simulink library "xpclib"  (Simulink 6.0)
settings: Solver=ode45  SolverMode=SingleTasking  StartTime=0.0  StopTime=10.0  RelTol=1e-3
values from neighbouring files (symbols this model uses):
  base = get_param( gcb, 'base' )    [maddiamondmm.m]    (also in maddiamondmm32.m; maddiamondmm32frame.m; maddsmm16at.m; malaim16.m = hex2dec(baseaddress(3:end)))
  data = ''    [mbwaudpmc.m]
  irq = params{3}    [mbaseserialmask.m]
  port = [0,1]    [canfifofilterutil.m]    (also in mbaseserialmask.m = str2num(get_param( gcb, 'port' )))
undefined symbols (not defined in the file or in its folder): CIO, devid, DIO24, genixlib, get, handlers, mbaseserialmask, mbwaudpmc, mdacbpcidas, mdiamondemeraldmask, mgenix, mmodemcontrol, mquamask, mrs232, msc150checks, mtargetboxleds, mtargetboxwatchdog, mxpccan, PCI, sizeof, vendid
libraries: xpclib x384, simulink x6
(part 5 of 7)

== system xpclib/RS232/Quatech/QSC-200/300 ==
  Modem Control : S-Function  InitFcn=mmodemcontrol(3)  FunctionName=modemcontrolqua  Parameters=slot, port, boardtype, rts, dtr, count  mask(QSC-200/300 Modem Control){port=1, rts=on, dtr=on, slot=-1}
      mask prompts: slot "PCI slot: (-1 for autosearch)"
      mask help:
      | QSC-200/300
      | Quatech
      | Modem Control
      mask init:
      | count = 0;
      | boardtype = 3;
      | [maskdisplay, count] = mmodemcontrol( 2, rts, dtr, boardtype, 0, 0 );
      | set_param( gcb, 'MaskDisplay', maskdisplay );
      mask Help: helpview(fullfile(docroot, 'mapfiles', 'xpc.map'), 'Quatech_MODEM_Control')
      mask StyleString: popup(1|2|3|4),checkbox,checkbox,edit
      mask Display: disp('QSC-200/300\nQuatech\nModem Control');port_label('input',1,'RTS');port_label('input',2,'DTR');
  Modem Status : S-Function  FunctionName=modemstatusqua  Parameters=slot, port, boardtype, cts, dsr, ring, dcd, count, sampletime  mask(Modem Status){port=1, cts=on, dsr=on, ring=on, dcd=on, sampletime=-1, slot=-1}
      mask prompts: ring "RI:"; slot "PCI slot: (-1 for autosearch)"
      mask help:
      | QSC-200/300
      | Quatech
      | Modem Status
      mask init:
      | count = 0;
      | boardtype = 3;
      | [maskdisplay, count] = mmodemstatus( 2, cts, dsr, ring, dcd, boardtype );
      | set_param( gcb, 'MaskDisplay', maskdisplay );
      mask Help: helpview(fullfile(docroot, 'mapfiles', 'xpc.map'), 'Quatech_MODEM_Status')
      mask StyleString: popup(1|2|3|4),checkbox,checkbox,checkbox,checkbox,edit,edit
      mask Display: disp('QSC-200/300\nQuatech\nModem Status');port_label('output',1,'CTS');port_label('output',2,'DSR');port_label('output',3,'RI');port_label('output',4,'DCD');
  QSC-200/300 Internal  blocks1 : Subsystem  PropExecContextAcrossSSBoundary=on
  "QSC-200/300 " : Subsystem  InitFcn=mquamask(3)  TreatAsAtomicUnit=on  PropExecContextAcrossSSBoundary=on  mask(RS422/485 Send Receive){group=Board Setup, port=1, irqnum=7, slot=-1, baud1=115200, parity1=None, ndata1=8, nstop1=1, fifomode1=64 deep, rlevel1=half full, onxmt1=None, xmtfifosize1=1024, xmtdatatype1=8 bit uint null terminated, rcvfifosize1=1024, rcvmaxread1=1024, rcvminread1=1, rcvusedelim1=on, rcvdelim1=13, rcvdatatype1=count+16 bit uint, rcvsampletime1=-1, baud2=115200, parity2=None, ndata2=8, nstop2=1, fifomode2=64 deep, rlevel2=half full, onxmt2=None, xmtfifosize2=1024, xmtdatatype2=8 bit uint null terminated, rcvfifosize2=1024, rcvmaxread2=1024, rcvminread2=1, rcvusedelim2=on, rcvdelim2=13, rcvdatatype2=count+16 bit uint, rcvsampletime2=-1, baud3=115200, parity3=None, ndata3=8, nstop3=1, fifomode3=64 deep, rlevel3=half full, onxmt3=None, xmtfifosize3=1024, xmtdatatype3=8 bit uint null terminated, rcvfifosize3=1024, rcvmaxread3=1024, rcvminread3=1, rcvusedelim3=on, rcvdelim3=13, rcvdatatype3=count+16 bit uint, rcvsampletime3=-1, buad4=115200, parity4=None, ndata4=8, nstop4=1, fifomode4=64 deep, rlevel4=half full, onxmt4=None, xmtfifosize4=1024, xmtdatatype4=8 bit uint null terminated, rcvfifosize4=1024, rcvmaxread4=1024, rcvminread4=1, rcvusedelim4=on, rcvdelim4=13, rcvdatatype4=count+16 bit uint, rcvsampletime4=-1}
      mask prompts: group "Parameter group:"; port "Port to modify:"; irqnum "IRQ number:"; baud1 "Baud rate:"; parity1 "Parity:"; ndata1 "Data bits:"; nstop1 "Stop bits:"; fifomode1 "Hardware fifo size:"; rlevel1 "Receive fifo interrupt level:"; onxmt1 "Assert on transmit:"; xmtfifosize1 "Transmit software fifo size:"; xmtdatatype1 "Transmit fifo data type:"; rcvfifosize1 "Receive software fifo size:"; rcvmaxread1 "Receive maximum read:"; rcvminread1 "Receive minimum read:"; rcvusedelim1 "Read to delimiter:"; rcvdelim1 "Delimiter:"; rcvdatatype1 "Receive data type:"; rcvsampletime1 "Receive SampleTime:"; baud2 "Baud rate:"; parity2 "Parity:"; ndata2 "Data bits:"; nstop2 "Stop bits:"; fifomode2 "Hardware fifo size:"; rlevel2 "Receive fifo interrupt level:"; onxmt2 "Assert on transmit:"; xmtfifosize2 "Transmit software fifo size:"; xmtdatatype2 "Transmit fifo data type:"; rcvfifosize2 "Receive software fifo size:"; rcvmaxread2 "Receive maximum read:"; rcvminread2 "Receive minimum read:"; rcvusedelim2 "Read to delimiter:"; rcvdelim2 "Delimiter:"; rcvdatatype2 "Receive data type:"; rcvsampletime2 "Receive SampleTime:"; baud3 "Baud rate:"; parity3 "Parity:"; ndata3 "Data bits:"; nstop3 "Stop bits:"; fifomode3 "Hardware fifo size:"; rlevel3 "Receive fifo interrupt level:"; onxmt3 "Assert on transmit:"; xmtfifosize3 "Transmit software fifo size:"; xmtdatatype3 "Transmit fifo data type:"; rcvfifosize3 "Receive software fifo size:"; rcvmaxread3 "Receive maximum read:"; rcvminread3 "Receive minimum read:"; rcvusedelim3 "Read to delimiter:"; rcvdelim3 "Delimiter:"; rcvdatatype3 "Receive data type:"; rcvsampletime3 "Receive SampleTime:"; buad4 "Baud rate:"; parity4 "Parity:"; ndata4 "Data bits:"; nstop4 "Stop bits:"; fifomode4 "Hardware fifo size:"; rlevel4 "Receive fifo interrupt level:"; onxmt4 "Assert on transmit:"; xmtfifosize4 "Transmit software fifo size:"; xmtdatatype4 "Transmit fifo data type:"; rcvfifosize4 "Receive software fifo size:"; rcvmaxread4 "Receive maximum read:"; rcvminread4 "Receive minimum read:"; rcvusedelim4 "Read to delimiter:"; rcvdelim4 "Delimiter:"; rcvdatatype4 "Receive data type:"; rcvsampletime4 "Receive SampleTime:"
      mask help:
      | QSC-200/300
      | Quatech
      | RS422/485 Send Receive Subsystem
      mask init:
      | brdslot = slot;
      | mqua2mask( 1, 4 );
      mask Help: helpview(fullfile(docroot, 'mapfiles', 'xpc.map'), 'Quatech_Subsystem')
      mask StyleString: popup(Board Setup|Basic Setup|Transmit Setup|Receive Setup),popup(1|2|3|4),edit,edit,popup(921600|460800|230400|115200|57600|38400|19200|9600|4800|2400|1200|600|300|110),popup(None|Even|Odd|Mark|Space),popup(5|6|7|8),popup(1|2),popup(64 deep|16 deep|1 deep),popup(1|quarter full|half full|almost full),popup(None|RTS|DTR),edit,popup(count+32 bit int|count+32 bit uint|count+16 bit int|count+16 bit uint|8 bit int null terminated|8 bit uint null terminated),edit,edit,edit,checkbox,edit,popup(count+32 bit int|count+32 bit uint|count+16 bit int|count+16 bit uint|8 bit int null terminated|8 bit uint null terminated),edit,popup(921600|460800|230400|115200|57600|38400|19200|9600|4800|2400|1200|600|300|110),popup(None|Even|Odd|Mark|Space),popup(5|6|7|8),popup(1|2),popup(64 deep|16 deep|1 deep),popup(1|quarter full|half full|almost full),popup(None|RTS|DTR),edit,popup(count+32 bit int|count+32 bit uint|count+16 bit int|count+16 bit uint|8 bit int null terminated|8 bit uint null terminated),edit,edit,edit,checkbox,edit,popup(count+32 bit int|count+32 bit uint|count+16 bit int|count+16 bit uint|8 bit int null terminated|8 bit uint null terminated),edit,popup(921600|460800|230400|115200|57600|38400|19200|9600|4800|2400|1200|600|300|110),popup(None|Even|Odd|Mark|Space),popup(5|6|7|8),popup(1|2),popup(64 deep|16 deep|1 deep),popup(1|quarter full|half full|almost full),popup(None|RTS|DTR),edit,popup(count+32 bit int|count+32 bit uint|count+16 bit int|count+16 bit uint|8 bit int null terminated|8 bit uint null terminated),edit,edit,edit,checkbox,edit,popup(count+32 bit int|count+32 bit uint|count+16 bit int|count+16 bit uint|8 bit int null terminated|8 bit uint null terminated),edit,popup(921600|460800|230400|115200|57600|38400|19200|9600|4800|2400|1200|600|300|110),popup(None|Even|Odd|Mark|Space),popup(5|6|7|8),popup(1|2),popup(64 deep|16 deep|1 deep),popup(1|quarter full|half full|almost full),popup(None|RTS|DTR),edit,popup(count+32 bit int|count+32 bit uint|count+16 bit int|count+16 bit uint|8 bit int null terminated|8 bit uint null terminated),edit,edit,edit,checkbox,edit,popup(count+32 bit int|count+32 bit uint|count+16 bit int|count+16 bit uint|8 bit int null terminated|8 bit uint null terminated),edit
      mask CallbackString:
      | mquamask( 2, 4 );
      | |mquamask( 2, 4 );||||||||||||||||||||||||||||||||||||||||||||||||||||||||||||||||||
      mask Display:
      | disp('QSC-200/300\n\nRS422/485\n\nSend Receive');
      | port_label( 'input', 1, 'XMT1' );
      | port_label( 'input', 2, 'XMT2' );
      | port_label( 'input', 3, 'XMT3' );
      | port_label( 'input', 4, 'XMT4' );
      | port_label( 'output', 1, 'RCV1' );
      | port_label( 'output', 2, 'RCV2' );
      | port_label( 'output', 3, 'RCV3' );
      | port_label( 'output', 4, 'RCV4' );

== system xpclib/RS232/Synchronous Mode/Send & Receive  ==
  In1 : Inport  LatchInput=off
  S-Function : S-Function  FunctionName=rs232_sendrec  Parameters=port,formatsend,formatrec,numb,ts
  Out1 : Outport
  wires:
  In1/1 -> S-Function/1
  S-Function/1 -> Out1/1

== system xpclib/CAN/Softing/CAN-AC2-104 SJA 1000/FIFO Mode ==
  "FIFO Read " : S-Function  FunctionName=canac2pcireceivef  Parameters=board, depth, status, sampletime  mask(canac2104readfifo){board=1, depth=1, status=off, sampletime=0.001}
      mask prompts: depth "FIFO read depth:"; status "Show status output port"; sampletime "Sample time:"
      mask help:
      | Softing
      | CAN-AC2-104
      | with SJA1000
      mask Help: helpview(fullfile(docroot, 'mapfiles', 'xpc.map'), 'Softing_CAN-AC2-104-SJA-1000_FIFO-Read')
      mask StyleString: popup(1|2|3),edit,checkbox,edit
      mask Display: disp(['CAN-AC2-104 B',num2str(board),'\nFIFO mode\nRead'])
  "FIFO Read Filter " : xpclib/CAN/Softing/CAN-AC2-PCI SJA 1000/FIFO Mode/FIFO Read Filter   portin=Any  direction=Exclude  ident=[]  identsel=Exclude
  "FIFO Read RCV Level " : S-Function  FunctionName=canac2readrcvfifolevel  Parameters=board, sampletime  mask(canac2readrcvfifolevel){board=1, sampletime=0.001}
      mask prompts: sampletime "Sample time:"
      mask help:
      | Softing
      | CAN-AC2-104
      | with SJA1000
      mask Help: helpview(fullfile(docroot, 'mapfiles', 'xpc.map'), 'Softing_CAN-AC2-104-SJA-1000_FIFO-Read-RCV-Level')
      mask StyleString: popup(1|2|3),edit
      mask Display: disp(['CAN-AC2-104 B',num2str(board),'\nFIFO mode\nRCV FIFO level'])
  "FIFO Read XMT Level " : S-Function  FunctionName=canac2readxmtfifolevel  Parameters=board, sampletime  mask(canac2readxmtfifolevel){board=1, sampletime=0.001}
      mask prompts: sampletime "Sample time:"
      mask help:
      | Softing
      | CAN-AC2-104
      | with SJA1000
      mask Help: helpview(fullfile(docroot, 'mapfiles', 'xpc.map'), 'Softing_CAN-AC2-104-SJA-1000_FIFO-Read-XMT-Level')
      mask StyleString: popup(1|2|3),edit
      mask Display: disp(['CAN-AC2-104 B',num2str(board),'\nFIFO mode\nXMT FIFO level'])
  "FIFO Reset RCV " : S-Function  FunctionName=canac2resetrcvfifo  Parameters=board, sampletime  mask(canac2resetrcvfifo){board=1, sampletime=0.001}
      mask prompts: sampletime "Sample time:"
      mask help:
      | Softing
      | CAN-AC2-104
      | with SJA1000
      mask Help: helpview(fullfile(docroot, 'mapfiles', 'xpc.map'), 'Softing_CAN-AC2-104-SJA-1000_FIFO-Reset-RCV')
      mask StyleString: popup(1|2|3),edit
      mask Display: disp(['CAN-AC2-104 B',num2str(board),'\nFIFO mode\nReset RCV FIFO'])
  "FIFO Reset XMT " : S-Function  FunctionName=canac2resetxmtfifo  Parameters=board, sampletime  mask(canac2resetxmtfifo){board=1, sampletime=0.001}
      mask prompts: sampletime "Sample time:"
      mask help:
      | Softing
      | CAN-AC2-104
      | with SJA1000
      mask Help: helpview(fullfile(docroot, 'mapfiles', 'xpc.map'), 'Softing_CAN-AC2-104-SJA-1000_FIFO-Reset-XMT')
      mask StyleString: popup(1|2|3),edit
      mask Display: disp(['CAN-AC2-104 B',num2str(board),'\nFIFO mode\nReset XMT FIFO'])
  "FIFO Setup " : S-Function  FunctionName=canac2104setupf  Parameters=can1UserBR, can2UserBR, initarray, termarray, ioBaseAddress, memBaseAddress, intNo, board, efdetection, acc1, acc2  mask(canac2104setupfifo){board=1, can1Baudrate=1 MBaud, can1UserBR=[1,1,4,3], acc1=[0,0,0,0], can2Baudrate=1 MBaud, can2UserBR=[1,1,4,3], acc2=[0,0,0,0], efdetection=off, init=[], term=[], ioBaseAddressL=0x300, memBaseAddressL=0xd0000, intNo=None}
      mask prompts: can1Baudrate "CAN 1 - baud rate:"; can1UserBR "CAN 1 - user defined baud rate:"; acc1 "CAN 1 - acceptance [StdMask, StdCode, ExtMask, ExtCode]:"; can2Baudrate "CAN 2 - baud rate:"; can2UserBR "CAN 2 - user defined baud rate:"; acc2 "CAN 2 - acceptance [StdMask, StdCode, ExtMask, ExtCode]:"; efdetection "Enable error frame detection"; init "Initialization command structure:"; term "Termination:"; ioBaseAddressL "I/O base address:"; memBaseAddressL "Memory base address:"; intNo "Interrupt line:"
      mask help:
      | Softing
      | CAN-AC2-104
      | with SJA1000
      mask init:
      | initarray=0;
      | termarray=0;
      | ioBaseAddress=768;
      | memBaseAddress=819200;
      | if strcmp(intNo,'None'), intNo='0'; end
      | intNo=str2num(intNo);
      | [can1UserBR, can2UserBR, initarray, termarray,ioBaseAddress,  memBaseAddress]= mxpccanf(1, can1Baudrate, can1UserBR, can2Baudrate, can2UserBR, init, term, ioBaseAddressL, memBaseAddressL, board);
      mask Help: helpview(fullfile(docroot, 'mapfiles', 'xpc.map'), 'Softing_CAN-AC2-104-SJA-1000_FIFO-Setup')
      mask StyleString: popup(1|2|3),popup(1 MBaud|800 kBaud|500 kBaud|250 kBaud|125 kBaud|100 kBaud|10 kBaud|User defined),edit,edit,popup(1 MBaud|800 kBaud|500 kBaud|250 kBaud|125 kBaud|100 kBaud|10 kBaud|User defined),edit,edit,checkbox,edit,edit,edit,edit,popup(None|5|9|10|11|12|15)
      mask Display: disp(['CAN-AC2-104 B',num2str(board),'\nFIFO: CAN 1 / CAN 2\nStandard / Extended'])
  "FIFO Write " : S-Function  FunctionName=canac2pcisendf  Parameters=board, status, sampletime  mask(canac2104writefifo){board=1, status=off, sampletime=0.001}
      mask prompts: status "Show status output port"; sampletime "Sample time:"
      mask help:
      | Softing
      | CAN-AC2-104
      | with SJA1000
      mask Help: helpview(fullfile(docroot, 'mapfiles', 'xpc.map'), 'Softing_CAN-AC2-104-SJA-1000_FIFO-Write')
      mask StyleString: popup(1|2|3),checkbox,edit
      mask Display: disp(['CAN-AC2-104 B',num2str(board),'\nFIFO mode\nWrite'])

== system xpclib/CAN/Softing/CAN-AC2-PCI SJA 1000/FIFO Mode ==
  "FIFO Read " : S-Function  FunctionName=canac2pcireceivef  Parameters=board, depth, status, sampletime  mask(canac2pcireadfifo){board=1, depth=1, status=off, sampletime=0.001}
      mask prompts: depth "FIFO read depth:"; status "Show status output port"; sampletime "Sample time:"
      mask help:
      | Softing
      | CAN-AC2-PCI
      | with SJA1000
      mask Help: helpview(fullfile(docroot, 'mapfiles', 'xpc.map'), 'Softing_CAN-AC2-PCI-SJA-1000_FIFO-Read')
      mask StyleString: popup(1|2|3),edit,checkbox,edit
      mask Display: disp(['CAN-AC2-PCI B',num2str(board),'\nFIFO mode\nRead'])
  "FIFO Read Filter " : S-Function  FunctionName=canfifofilter  Parameters=port, ctype, ident, identsel-1  mask(canrcvfifofilter){portin=Any, ctypein=, direction=Exclude, ident=[], identsel=Exclude}
      mask prompts: portin "CAN port:"; ctypein "Message type command (SDF SRF EDF ERF EF NE CBS):"; direction "Message type selection mode:"; ident "Identifier(s):"; identsel "Identifier selection mode:"
      mask help:
      | CAN
      | FIFO Read Filter
      mask init:
      | [port, ctype]= canfifofilterutil(portin, ctypein, direction-1);
      | if portin==1, portd='any'; end
      | if portin==2, portd='1'; end
      | if portin==3, portd='2'; end
      | if direction==1, dird='+: '; end
      | if direction==2, dird='-: '; end
      | if identsel==1, seld='+: '; end
      | if identsel==2, seld='-: '; end
      | identd= xpcdarray2str(ident);
      mask Help: helpview(fullfile(docroot, 'mapfiles', 'xpc.map'), 'Softing_CAN-AC2-PCI-SJA-1000_FIFO-Read-Filter')
      mask StyleString: popup(Any|1|2),edit,popup(Include|Exclude),edit,popup(Include|Exclude)
      mask Display: disp(['Port: ',portd,'\n',dird,ctypein,'\n',seld,identd]);
  "FIFO Read RCV Level " : S-Function  FunctionName=canac2readrcvfifolevel  Parameters=board, sampletime  mask(canac2readrcvfifolevel){board=1, sampletime=0.001}
      mask prompts: sampletime "Sample time:"
      mask help:
      | Softing
      | CAN-AC2-PCI
      | with SJA1000
      mask Help: helpview(fullfile(docroot, 'mapfiles', 'xpc.map'), 'Softing_CAN-AC2-PCI-SJA-1000_FIFO-Read-RCV-Level')
      mask StyleString: popup(1|2|3),edit
      mask Display: disp(['CAN-AC2-PCI B',num2str(board),'\nFIFO mode\nRCV FIFO level'])
  "FIFO Read XMT Level " : S-Function  FunctionName=canac2readxmtfifolevel  Parameters=board, sampletime  mask(canac2readxmtfifolevel){board=1, sampletime=0.001}
      mask prompts: sampletime "Sample time:"
      mask help:
      | Softing
      | CAN-AC2-PCI
      | with SJA1000
      mask Help: helpview(fullfile(docroot, 'mapfiles', 'xpc.map'), 'Softing_CAN-AC2-PCI-SJA-1000_FIFO-Read-XMT-Level')
      mask StyleString: popup(1|2|3),edit
      mask Display: disp(['CAN-AC2-PCI B',num2str(board),'\nFIFO mode\nXMT FIFO level'])
  "FIFO Reset RCV " : S-Function  FunctionName=canac2resetrcvfifo  Parameters=board, sampletime  mask(canac2resetrcvfifo){board=1, sampletime=0.001}
      mask prompts: sampletime "Sample time:"
      mask help:
      | Softing
      | CAN-AC2-PCI
      | with SJA1000
      mask Help: helpview(fullfile(docroot, 'mapfiles', 'xpc.map'), 'Softing_CAN-AC2-PCI-SJA-1000_FIFO-Reset-RCV')
      mask StyleString: popup(1|2|3),edit
      mask Display: disp(['CAN-AC2-PCI B',num2str(board),'\nFIFO mode\nReset RCV FIFO'])
  "FIFO Reset XMT " : S-Function  FunctionName=canac2resetxmtfifo  Parameters=board, sampletime  mask(canac2resetxmtfifo){board=1, sampletime=0.001}
      mask prompts: sampletime "Sample time:"
      mask help:
      | Softing
      | CAN-AC2-PCI
      | with SJA1000
      mask Help: helpview(fullfile(docroot, 'mapfiles', 'xpc.map'), 'Softing_CAN-AC2-PCI-SJA-1000_FIFO-Reset-XMT')
      mask StyleString: popup(1|2|3),edit
      mask Display: disp(['CAN-AC2-PCI B',num2str(board),'\nFIFO mode\nReset XMT FIFO'])
  "FIFO Setup " : S-Function  FunctionName=canac2pcisetupf  Parameters=can1UserBR, can2UserBR, initarray, termarray, ioBaseAddress, memBaseAddress, intNo, board, can1bus, can2bus, efdetection, acc1, acc2  mask(canac2pcisetupfifo){board=1, can1bus=Highspeed (ISO 11898), can1Baudrate=1 MBaud, can1UserBR=[1,1,4,3], acc1=[0,0,0,0], can2bus=Highspeed (ISO 11898), can2Baudrate=1 MBaud, can2UserBR=[1,1,4,3], acc2=[0,0,0,0], efdetection=off, init=[], term=[], ioBaseAddress=-1}
      mask prompts: can1bus "CAN 1 - physical bus:"; can1Baudrate "CAN 1 - baud rate:"; can1UserBR "CAN 1 - user defined baud rate:"; acc1 "CAN 1 - acceptance [StdMask, StdCode, ExtMask, ExtCode]:"; can2bus "CAN 2 - physical bus:"; can2Baudrate "CAN 2 - baud rate:"; can2UserBR "CAN 2 - user defined baud rate:"; acc2 "CAN 2 - acceptance [StdMask, StdCode, ExtMask, ExtCode]:"; efdetection "Enable error frame detection"; init "Initialization command structure:"; term "Termination:"; ioBaseAddress "PCI slot (-1: autosearch):"
      mask help:
      | Softing
      | CAN-AC2-PCI
      | with SJA1000
      mask init:
      | can1str='';can2str='';
      | if can1bus==2, can1str=' LS'; end;if can2bus==2, can2str=' LS'; end;
      | initarray=0;
      | termarray=0;
      | ioBaseAddressL='0'; memBaseAddressL='0';
      | memBaseAddress=819200;
      | intNo=0;
      | [can1UserBR, can2UserBR, initarray, termarray]= mxpccanf(2, can1Baudrate, can1UserBR, can2Baudrate, can2UserBR, init, term, ioBaseAddressL, memBaseAddressL, board);
      | ;
      mask Help: helpview(fullfile(docroot, 'mapfiles', 'xpc.map'), 'Softing_CAN-AC2-PCI-SJA-1000_FIFO-Setup')
      mask StyleString: popup(1|2|3),popup(Highspeed (ISO 11898) |Lowspeed (requires LS module)),popup(1 MBaud|800 kBaud|500 kBaud|250 kBaud|125 kBaud|100 kBaud|10 kBaud|User defined),edit,edit,popup(Highspeed (ISO 11898) |Lowspeed (requires LS module)),popup(1 MBaud|800 kBaud|500 kBaud|250 kBaud|125 kBaud|100 kBaud|10 kBaud|User defined),edit,edit,checkbox,edit,edit,edit
      mask Display: disp(['CAN-AC2-PCI B',num2str(board),'\nFIFO: CAN 1',can1str,' / CAN 2',can2str,'\nStandard / Extended'])
  "FIFO Write " : S-Function  FunctionName=canac2pcisendf  Parameters=board, status, sampletime  mask(canac2pciwritefifo){board=1, status=off, sampletime=0.001}
      mask prompts: status "Show status output port"; sampletime "Sample time:"
      mask help:
      | Softing
      | CAN-AC2-PCI
      | with SJA1000
      mask Help: helpview(fullfile(docroot, 'mapfiles', 'xpc.map'), 'Softing_CAN-AC2-PCI-SJA-1000_FIFO-Write')
      mask StyleString: popup(1|2|3),checkbox,edit
      mask Display: disp(['CAN-AC2-PCI B',num2str(board),'\nFIFO mode\nWrite'])

== system xpclib/RS232/Diamond/Emerald-MM /Diamond Emerald-MM ==
  "Enable TX " : S-Function  FunctionName=sertxenableemeraldmm  Parameters=addr  mask(Enable TX Int){addr=-1}
      mask prompts: addr "Base address:"
      mask help:
      | Diamond Emerald
      | Enable TX Interrupt
      mask init:
      | addr = hex2dec( addr(3:end) );
      mask Help: helpview(fullfile(docroot, 'mapfiles', 'xpc.map'), 'Baseboard_Enable_Int')
      mask Display:
      | disp('Diamond\nEmerald-MM\nEnable TX int');
      | port_label('input', 1, 'E');
  Filter Int Reason : S-Function  FunctionName=filterserint  Parameters=port, value  mask(Interrupt Source Filter){port=1, value=Receive data}
      mask prompts: value "Filter value:"
      mask help:
      | Diamond Emerald-MM
      | Interrupt Source Filter
      mask Help: helpview(fullfile(docroot, 'mapfiles', 'xpc.map'), 'Baseboard_Filter_Ints')
      mask StyleString: popup(1|2|3|4),popup(Receive data|Transmitter empty|Modem status change)
      mask Display:
      | disp('Diamond\nEmerald\nFilter');
      | port_label('input', 1, 'S' );
      | port_label('output', 1, 'E' );
  Read HW FIFO : S-Function  FunctionName=serreademeraldmm  Parameters=addr, flush  mask(Read Data Port){flush=on, addr=0}
      mask prompts: flush "Flush HW FIFO on startup"; addr "Base address:"
      mask help:
      | Diamond Emerald-MM
      | Read Data Port
      mask init:
      | addr = hex2dec( addr(3:end) );
      mask Help: helpview(fullfile(docroot, 'mapfiles', 'xpc.map'), 'Baseboard_Read_HW')
      mask Display:
      | disp('Diamond\nEmerald-MM\nRead Data Port');
      | port_label('input', 1, 'E');
      | port_label('output', 1, 'D');
  Read Int Status : S-Function  FunctionName=iqueryemeraldmm  Parameters=addr1, addr2, addr3, addr4, intstat  mask(Interrupt Query){addr1=0, addr2=0, addr3=0, addr4=0, intstat=0}
      mask prompts: addr1 "First port address:"; addr2 "Second port address:"; addr3 "Third port address:"; addr4 "Fourth port address:"; intstat "Interrupt status address"
      mask help:
      | Diamond Emerald-MM
      | Interrupt Query
      mask init:
      | addr1 = hex2dec( addr1(3:end) );
      | addr2 = hex2dec( addr2(3:end) );
      | addr3 = hex2dec( addr3(3:end) );
      | addr4 = hex2dec( addr4(3:end) );
      | intstat = hex2dec( intstat(3:end) );
      mask Help: helpview(fullfile(docroot, 'mapfiles', 'xpc.map'), 'Baseboard_Interrupt_Query')
      mask Display:
      | disp('Diamond\nEmerald-MM\nInt Status');
      | port_label('output', 1, 'S' );
  Setup : S-Function  FunctionName=sersetupemeraldmm  Parameters=addr, baud, width, nstop, parity, fmode, ctsmode, rlevel  mask(setup){baud=115200, width=8, nstop=1, parity=None, fmode=16 deep, rlevel=half full, ctsmode=on, addr=0}
      mask prompts: baud "Baud rate:"; width "Number of data bits:"; nstop "Number of stop bits:"; fmode "Fifo mode:"; rlevel "Receive trigger level:"; ctsmode "Enable auto RTS/CTS"; addr "Base address:"
      mask help:
      | Diamond Emerald-MM
      | Serial
      | Setup
      mask init:
      | addr = hex2dec( addr(3:end) );
      mask Help: helpview(fullfile(docroot, 'mapfiles', 'xpc.map'), 'Baseboard_Setup')
      mask StyleString: popup(115200|57600|38400|19200|9600|4800|2400|1200|600|300|110),popup(5|6|7|8),popup(1|2),popup(None|Even|Odd|Mark|Space),popup(64 deep|16 deep|1 deep),popup(1|quarter full|half full|almost full),checkbox,edit
      mask Display: disp('Diamond\nEmerald-MM\nSetup');
  Write HW FIFO : S-Function  FunctionName=serwriteemeraldmm  Parameters=addr  mask(Write Data Port){addr=-1}
      mask prompts: addr "Base address:"
      mask help:
      | Diamond Emerald-MM
      | Write Data Port
      mask init:
      | addr = hex2dec( addr(3:end) );
      mask Help: helpview(fullfile(docroot, 'mapfiles', 'xpc.map'), 'Baseboard_Write_HW')
      mask Display:
      | disp('Diamond\nEmerald-MM\nWrite Data Port');
      | port_label('input', 1, 'D');
      | port_label('input', 2, 'E');

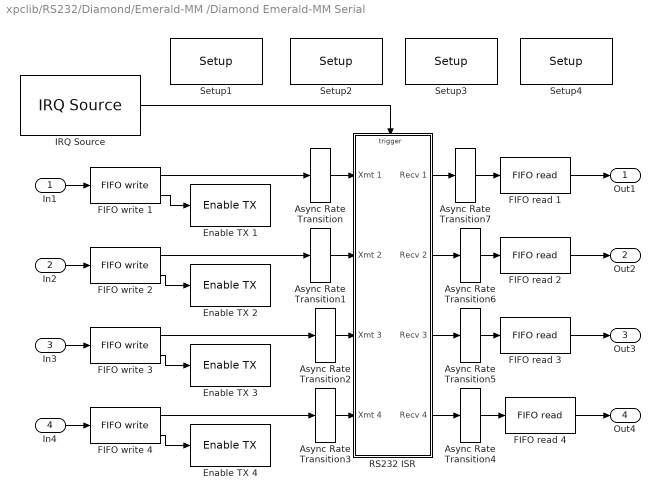
== system xpclib/RS232/Diamond/Emerald-MM /Diamond Emerald-MM Serial ==
  In1 : Inport  LatchInput=off
  In2 : Inport  Port=2  LatchInput=off
  In3 : Inport  Port=3  LatchInput=off
  In4 : Inport  Port=4  LatchInput=off
  Async Rate Transition{,1..7} (8 alike) : xpclib/Asynchronous Event/Async Rate Transition  sample_time=-1
  Enable TX 1 : xpclib/RS232/Diamond/Emerald-MM /Diamond Emerald-MM/Enable TX   addr=baddr1
  Enable TX 2 : xpclib/RS232/Diamond/Emerald-MM /Diamond Emerald-MM/Enable TX   addr=baddr2
  Enable TX 3 : xpclib/RS232/Diamond/Emerald-MM /Diamond Emerald-MM/Enable TX   addr=baddr3
  Enable TX 4 : xpclib/RS232/Diamond/Emerald-MM /Diamond Emerald-MM/Enable TX   addr=baddr4
  FIFO read {1..4} (4 alike) : xpclib/RS232/FIFO read   maxsize=1024  minsize=1  usedelimiter=on  delimiter=13  outputtype=count+16 bit uint  enable=off  enableout=off  sampletime=-1
  FIFO write 1 : xpclib/RS232/FIFO write   size=1024  inputtype=8 bit uint null terminated  present=on  sampletime=-1  id=XMT channel 1, IRQ 7
  FIFO write 2 : xpclib/RS232/FIFO write   size=1024  inputtype=8 bit uint null terminated  present=on  sampletime=-1  id=XMT channel 2, IRQ 7
  FIFO write 3 : xpclib/RS232/FIFO write   size=1024  inputtype=8 bit uint null terminated  present=on  sampletime=-1  id=XMT channel 3, IRQ 7
  FIFO write 4 : xpclib/RS232/FIFO write   size=1024  inputtype=8 bit uint null terminated  present=on  sampletime=-1  id=XMT channel 4, IRQ 7
  IRQ Source : xpclib/Asynchronous Event/IRQ Source  irqNo=7  preempt=off  b_type=None/Other  slot=-1
  RS232 ISR : Subsystem  TreatAsAtomicUnit=on  PropExecContextAcrossSSBoundary=on  mask(RS232 ISR){addr1=baddr1, addr2=baddr2, addr3=baddr3, addr4=baddr4, intstat=istat}
      mask prompts: addr1 "First channel address:"; addr2 "Second channel address:"; addr3 "Third channel address:"; addr4 "Fourth channel address:"; intstat "Status register address:"
      mask help:
      | Baseboard Serial
      | Interrupt Service Routine
      mask init:
      | baddr1 = addr1;
      | baddr2 = addr2;
      | baddr3 = addr3;
      | baddr4 = addr4;
      | istat = intstat;
      mask Display:
      | disp('Diamond\nEmerald\nSerial\nISR');
      | port_label('input', 1, 'XMT1');
      | port_label('input', 2, 'XMT2');
      | port_label('input', 3, 'XMT3');
      | port_label('input', 4, 'XMT4');
      | port_label('output', 1, 'RCV1');
      | port_label('output', 2, 'RCV2');
      | port_label('output', 3, 'RCV3');
      | port_label('output', 4, 'RCV4');
  Setup1 : xpclib/RS232/Diamond/Emerald-MM /Diamond Emerald-MM/Setup  baud=115200  width=8  nstop=1  parity=None  fmode=16 deep  rlevel=half full  ctsmode=on  addr=baddr1
  Setup2 : xpclib/RS232/Diamond/Emerald-MM /Diamond Emerald-MM/Setup  baud=115200  width=8  nstop=1  parity=None  fmode=16 deep  rlevel=half full  ctsmode=on  addr=baddr2
  Setup3 : xpclib/RS232/Diamond/Emerald-MM /Diamond Emerald-MM/Setup  baud=115200  width=8  nstop=1  parity=None  fmode=16 deep  rlevel=half full  ctsmode=on  addr=baddr3
  Setup4 : xpclib/RS232/Diamond/Emerald-MM /Diamond Emerald-MM/Setup  baud=115200  width=8  nstop=1  parity=None  fmode=16 deep  rlevel=half full  ctsmode=on  addr=baddr4
  Out1 : Outport
  Out2 : Outport  Port=2
  Out3 : Outport  Port=3
  Out4 : Outport  Port=4
  wires:
  FIFO write 4/2 -> Enable TX 4/1
  FIFO write 3/2 -> Enable TX 3/1
  FIFO write 2/2 -> Enable TX 2/1
  RS232 ISR/4(Recv 4) -> Async Rate Transition4/1
  RS232 ISR/3(Recv 3) -> Async Rate Transition5/1
  Async Rate Transition3/1 -> RS232 ISR/4(Xmt 4)
  Async Rate Transition2/1 -> RS232 ISR/3(Xmt 3)
  FIFO write 3/1 -> Async Rate Transition2/1
  FIFO write 4/1 -> Async Rate Transition3/1
  Async Rate Transition4/1 -> FIFO read 4/1
  Async Rate Transition5/1 -> FIFO read 3/1
  FIFO read 4/1 -> Out4/1
  FIFO read 3/1 -> Out3/1
  In3/1 -> FIFO write 3/1
  In4/1 -> FIFO write 4/1
  Async Rate Transition1/1 -> RS232 ISR/2(Xmt 2)
  RS232 ISR/2(Recv 2) -> Async Rate Transition6/1
  RS232 ISR/1(Recv 1) -> Async Rate Transition7/1
  FIFO read 2/1 -> Out2/1
  Async Rate Transition6/1 -> FIFO read 2/1
  FIFO read 1/1 -> Out1/1
  Async Rate Transition7/1 -> FIFO read 1/1
  In2/1 -> FIFO write 2/1
  FIFO write 2/1 -> Async Rate Transition1/1
  In1/1 -> FIFO write 1/1
  FIFO write 1/1 -> Async Rate Transition/1
  Async Rate Transition/1 -> RS232 ISR/1(Xmt 1)
  IRQ Source/1 -> RS232 ISR/Trigger
  FIFO write 1/2 -> Enable TX 1/1

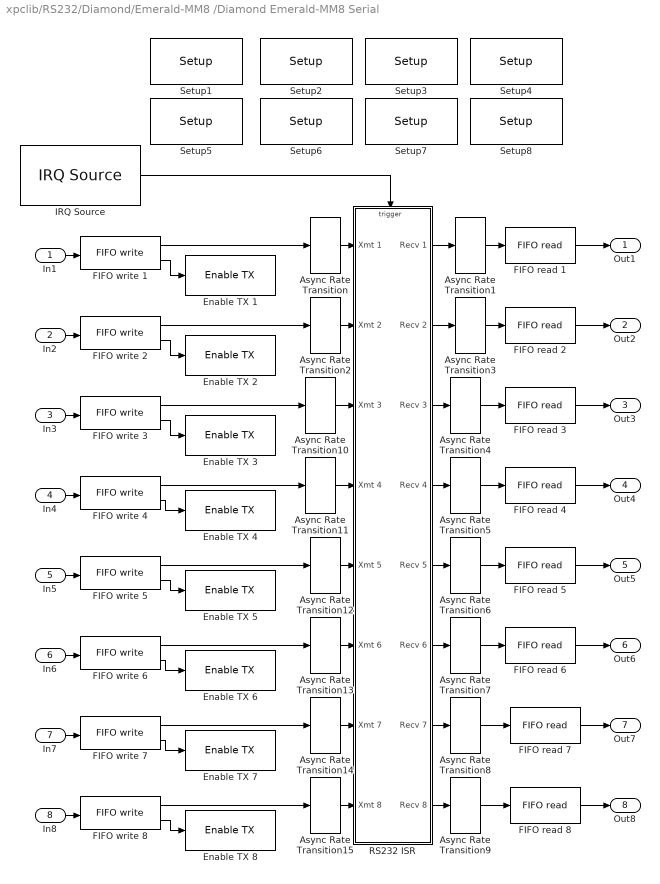
== system xpclib/RS232/Diamond/Emerald-MM8 /Diamond Emerald-MM8 Serial ==
  In1 : Inport  LatchInput=off
  In2 : Inport  Port=2  LatchInput=off
  In3 : Inport  Port=3  LatchInput=off
  In4 : Inport  Port=4  LatchInput=off
  In5 : Inport  Port=5  LatchInput=off
  In6 : Inport  Port=6  LatchInput=off
  In7 : Inport  Port=7  LatchInput=off
  In8 : Inport  Port=8  LatchInput=off
  Async Rate Transition{,1..15} (16 alike) : xpclib/Asynchronous Event/Async Rate Transition  sample_time=-1
  Enable TX 1 : xpclib/RS232/Diamond/Emerald-MM8 /Diamond Emerald-MM8 /Enable TX   addr=baddr1
  Enable TX 2 : xpclib/RS232/Diamond/Emerald-MM8 /Diamond Emerald-MM8 /Enable TX   addr=baddr2
  Enable TX 3 : xpclib/RS232/Diamond/Emerald-MM8 /Diamond Emerald-MM8 /Enable TX   addr=baddr3
  Enable TX 4 : xpclib/RS232/Diamond/Emerald-MM8 /Diamond Emerald-MM8 /Enable TX   addr=baddr4
  Enable TX 5 : xpclib/RS232/Diamond/Emerald-MM8 /Diamond Emerald-MM8 /Enable TX   addr=baddr5
  Enable TX 6 : xpclib/RS232/Diamond/Emerald-MM8 /Diamond Emerald-MM8 /Enable TX   addr=baddr6
  Enable TX 7 : xpclib/RS232/Diamond/Emerald-MM8 /Diamond Emerald-MM8 /Enable TX   addr=baddr7
  Enable TX 8 : xpclib/RS232/Diamond/Emerald-MM8 /Diamond Emerald-MM8 /Enable TX   addr=baddr8
  FIFO read {1..8} (8 alike) : xpclib/RS232/FIFO read   maxsize=1024  minsize=1  usedelimiter=on  delimiter=13  outputtype=count+16 bit uint  enable=off  enableout=off  sampletime=-1
  FIFO write 1 : xpclib/RS232/FIFO write   size=1024  inputtype=8 bit uint null terminated  present=on  sampletime=-1  id=XMT channel 1, IRQ 5
  FIFO write 2 : xpclib/RS232/FIFO write   size=1024  inputtype=8 bit uint null terminated  present=on  sampletime=-1  id=XMT channel 2, IRQ 5
  FIFO write 3 : xpclib/RS232/FIFO write   size=1024  inputtype=8 bit uint null terminated  present=on  sampletime=-1  id=XMT channel 3, IRQ 5
  FIFO write 4 : xpclib/RS232/FIFO write   size=1024  inputtype=8 bit uint null terminated  present=on  sampletime=-1  id=XMT channel 4, IRQ 5
  FIFO write 5 : xpclib/RS232/FIFO write   size=1024  inputtype=8 bit uint null terminated  present=on  sampletime=-1  id=XMT channel 5, IRQ 5
  FIFO write 6 : xpclib/RS232/FIFO write   size=1024  inputtype=8 bit uint null terminated  present=on  sampletime=-1  id=XMT channel 6, IRQ 5
  FIFO write 7 : xpclib/RS232/FIFO write   size=1024  inputtype=8 bit uint null terminated  present=on  sampletime=-1  id=XMT channel 7, IRQ 5
  FIFO write 8 : xpclib/RS232/FIFO write   size=1024  inputtype=8 bit uint null terminated  present=on  sampletime=-1  id=XMT channel 8, IRQ 5
  IRQ Source : xpclib/Asynchronous Event/IRQ Source  irqNo=5  preempt=off  b_type=None/Other  slot=-1
  RS232 ISR : Subsystem  TreatAsAtomicUnit=on  PropExecContextAcrossSSBoundary=on  mask(RS232 ISR){addr1=baddr1, addr2=baddr2, addr3=baddr3, addr4=baddr4, intstat=istat}
      mask prompts: addr1 "First channel address:"; addr2 "Second channel address:"; addr3 "Third channel address:"; addr4 "Fourth channel address:"; intstat "Status register address:"
      mask help:
      | Baseboard Serial
      | Interrupt Service Routine
      mask init:
      | baddr1 = addr1;
      | baddr2 = addr2;
      | baddr3 = addr3;
      | baddr4 = addr4;
      | istat = intstat;
      mask Display:
      | disp('Diamond\nEmerald\nSerial\nISR');
      | port_label('input', 1, 'XMT1');
      | port_label('input', 2, 'XMT2');
      | port_label('input', 3, 'XMT3');
      | port_label('input', 4, 'XMT4');
      | port_label('input', 5, 'XMT5');
      | port_label('input', 6, 'XMT6');
      | port_label('input', 7, 'XMT7');
      | port_label('input', 8, 'XMT8');
      | port_label('output', 1, 'RCV1');
      | port_label('output', 2, 'RCV2');
      | port_label('output', 3, 'RCV3');
      | port_label('output', 4, 'RCV4');
      | port_label('output', 5, 'RCV5');
      | port_label('output', 6, 'RCV6');
      | port_label('output', 7, 'RCV7');
      | port_label('output', 8, 'RCV8');
  Setup1 : xpclib/RS232/Diamond/Emerald-MM8 /Diamond Emerald-MM8 /Setup  baud=115200  width=8  nstop=1  parity=None  fmode=16 deep  rlevel=1  ctsmode=on  addr=baddr1  irq=irqnum
  Setup2 : xpclib/RS232/Diamond/Emerald-MM8 /Diamond Emerald-MM8 /Setup  baud=115200  width=8  nstop=1  parity=None  fmode=16 deep  rlevel=1  ctsmode=on  addr=baddr2  irq=irqnum
  Setup3 : xpclib/RS232/Diamond/Emerald-MM8 /Diamond Emerald-MM8 /Setup  baud=115200  width=8  nstop=1  parity=None  fmode=16 deep  rlevel=1  ctsmode=on  addr=baddr3  irq=irqnum
  Setup4 : xpclib/RS232/Diamond/Emerald-MM8 /Diamond Emerald-MM8 /Setup  baud=115200  width=8  nstop=1  parity=None  fmode=16 deep  rlevel=1  ctsmode=on  addr=baddr4  irq=irqnum
  Setup5 : xpclib/RS232/Diamond/Emerald-MM8 /Diamond Emerald-MM8 /Setup  baud=115200  width=8  nstop=1  parity=None  fmode=16 deep  rlevel=1  ctsmode=on  addr=baddr5  irq=irqnum
  Setup6 : xpclib/RS232/Diamond/Emerald-MM8 /Diamond Emerald-MM8 /Setup  baud=115200  width=8  nstop=1  parity=None  fmode=16 deep  rlevel=1  ctsmode=on  addr=baddr6  irq=irqnum
  Setup7 : xpclib/RS232/Diamond/Emerald-MM8 /Diamond Emerald-MM8 /Setup  baud=115200  width=8  nstop=1  parity=None  fmode=16 deep  rlevel=1  ctsmode=on  addr=baddr7  irq=irqnum
  Setup8 : xpclib/RS232/Diamond/Emerald-MM8 /Diamond Emerald-MM8 /Setup  baud=115200  width=8  nstop=1  parity=None  fmode=16 deep  rlevel=1  ctsmode=on  addr=baddr8  irq=irqnum
  Out1 : Outport
  Out2 : Outport  Port=2
  Out3 : Outport  Port=3
  Out4 : Outport  Port=4
  Out5 : Outport  Port=5
  Out6 : Outport  Port=6
  Out7 : Outport  Port=7
  Out8 : Outport  Port=8
  wires:
  FIFO write 2/1 -> Async Rate Transition2/1
  RS232 ISR/8(Recv 8) -> Async Rate Transition9/1
  RS232 ISR/7(Recv 7) -> Async Rate Transition8/1
  RS232 ISR/6(Recv 6) -> Async Rate Transition7/1
  RS232 ISR/5(Recv 5) -> Async Rate Transition6/1
  Async Rate Transition15/1 -> RS232 ISR/8(Xmt 8)
  Async Rate Transition14/1 -> RS232 ISR/7(Xmt 7)
  Async Rate Transition13/1 -> RS232 ISR/6(Xmt 6)
  Async Rate Transition12/1 -> RS232 ISR/5(Xmt 5)
  FIFO read 8/1 -> Out8/1
  Async Rate Transition9/1 -> FIFO read 8/1
  FIFO read 7/1 -> Out7/1
  Async Rate Transition8/1 -> FIFO read 7/1
  FIFO read 6/1 -> Out6/1
  Async Rate Transition7/1 -> FIFO read 6/1
  FIFO read 5/1 -> Out5/1
  Async Rate Transition6/1 -> FIFO read 5/1
  FIFO write 8/2 -> Enable TX 8/1
  FIFO write 8/1 -> Async Rate Transition15/1
  In8/1 -> FIFO write 8/1
  FIFO write 7/2 -> Enable TX 7/1
  FIFO write 7/1 -> Async Rate Transition14/1
  In7/1 -> FIFO write 7/1
  FIFO write 6/2 -> Enable TX 6/1
  FIFO write 6/1 -> Async Rate Transition13/1
  In6/1 -> FIFO write 6/1
  FIFO write 5/2 -> Enable TX 5/1
  FIFO write 5/1 -> Async Rate Transition12/1
  In5/1 -> FIFO write 5/1
  FIFO write 4/2 -> Enable TX 4/1
  FIFO write 3/2 -> Enable TX 3/1
  FIFO write 2/2 -> Enable TX 2/1
  FIFO write 1/2 -> Enable TX 1/1
  RS232 ISR/4(Recv 4) -> Async Rate Transition5/1
  RS232 ISR/3(Recv 3) -> Async Rate Transition4/1
  Async Rate Transition11/1 -> RS232 ISR/4(Xmt 4)
  Async Rate Transition10/1 -> RS232 ISR/3(Xmt 3)
  FIFO write 3/1 -> Async Rate Transition10/1
  FIFO write 4/1 -> Async Rate Transition11/1
  Async Rate Transition5/1 -> FIFO read 4/1
  Async Rate Transition4/1 -> FIFO read 3/1
  FIFO read 4/1 -> Out4/1
  FIFO read 3/1 -> Out3/1
  In3/1 -> FIFO write 3/1
  In4/1 -> FIFO write 4/1
  Async Rate Transition2/1 -> RS232 ISR/2(Xmt 2)
  RS232 ISR/2(Recv 2) -> Async Rate Transition3/1
  RS232 ISR/1(Recv 1) -> Async Rate Transition1/1
  FIFO read 2/1 -> Out2/1
  Async Rate Transition3/1 -> FIFO read 2/1
  FIFO read 1/1 -> Out1/1
  Async Rate Transition1/1 -> FIFO read 1/1
  In2/1 -> FIFO write 2/1
  In1/1 -> FIFO write 1/1
  FIFO write 1/1 -> Async Rate Transition/1
  Async Rate Transition/1 -> RS232 ISR/1(Xmt 1)
  IRQ Source/1 -> RS232 ISR/Trigger

== system xpclib/RS232/Diamond/Emerald-MM8 /Diamond Emerald-MM8  ==
  "Enable TX " : S-Function  FunctionName=sertxenableemeraldmm  Parameters=addr  mask(Enable TX Int){addr='0x208'}
      mask prompts: addr "Base address:"
      mask help:
      | Diamond Emerald
      | Enable TX Interrupt
      mask init:
      | addr = hex2dec( addr(3:end) );
      mask Help: helpview(fullfile(docroot, 'mapfiles', 'xpc.map'), 'Baseboard_Enable_Int')
      mask Display:
      | disp('Diamond\nEmerald-MM8\nEnable TX int');
      | port_label('input', 1, 'E');
  Filter Int Reason : S-Function  FunctionName=filterserint  Parameters=port, value  mask(Interrupt Source Filter){port=1, value=Receive data}
      mask prompts: value "Filter value:"
      mask help:
      | Diamond Emerald-MM
      | Interrupt Source Filter
      mask Help: helpview(fullfile(docroot, 'mapfiles', 'xpc.map'), 'Baseboard_Filter_Ints')
      mask StyleString: popup(1|2|3|4|5|6|7|8),popup(Receive data|Transmitter empty|Modem status change)
      mask Display:
      | disp('Diamond\nEmerald-MM8\nFilter');
      | port_label('input', 1, 'S' );
      | port_label('output', 1, 'E' );
  Read HW FIFO : S-Function  FunctionName=serreademeraldmm  Parameters=addr, flush  mask(Read Data Port){flush=on, addr=0}
      mask prompts: flush "Flush HW FIFO on startup"; addr "Base address:"
      mask help:
      | Diamond Emerald-MM
      | Read Data Port
      mask init:
      | addr = hex2dec( addr(3:end) );
      mask Help: helpview(fullfile(docroot, 'mapfiles', 'xpc.map'), 'Baseboard_Read_HW')
      mask Display:
      | disp('Diamond\nEmerald-MM8\nRead Data Port');
      | port_label('input', 1, 'E');
      | port_label('output', 1, 'D');
  Read Int Status : S-Function  FunctionName=iqueryemeraldmm8  Parameters=addr1, addr2, addr3, addr4, addr5, addr6, addr7, addr8, intstat  mask(Interrupt Query){addr1=0, addr2=0, addr3=0, addr4=0, addr5=0, addr6=0, addr7=0, addr8=0, intstat=0}
      mask prompts: addr1 "First port address:"; addr2 "Second port address:"; addr3 "Third port address:"; addr4 "Fourth port address:"; addr5 "Fifth port address:"; addr6 "Sixth port address:"; addr7 "Seventh port address:"; addr8 "Eighth port address:"; intstat "Interrupt status address"
      mask help:
      | Diamond Emerald-MM8
      | Interrupt Query
      mask init:
      | addr1 = hex2dec( addr1(3:end) );
      | addr2 = hex2dec( addr2(3:end) );
      | addr3 = hex2dec( addr3(3:end) );
      | addr4 = hex2dec( addr4(3:end) );
      | addr5 = hex2dec( addr5(3:end) );
      | addr6 = hex2dec( addr6(3:end) );
      | addr7 = hex2dec( addr7(3:end) );
      | addr8 = hex2dec( addr8(3:end) );
      | intstat = hex2dec( intstat(3:end) );
      mask Help: helpview(fullfile(docroot, 'mapfiles', 'xpc.map'), 'Baseboard_Interrupt_Query')
      mask Display:
      | disp('Diamond\nEmerald-MM8\nInt Status');
      | port_label('output', 1, 'S' );
  Setup : S-Function  FunctionName=sersetupemeraldmm8  Parameters=addr, irq, baud, width, nstop, parity, fmode, ctsmode, rlevel  mask(setup){baud=115200, width=8, nstop=1, parity=None, fmode=16 deep, rlevel=half full, ctsmode=on, addr=0, irq=0}
      mask prompts: baud "Baud rate:"; width "Number of data bits:"; nstop "Number of stop bits:"; fmode "Fifo mode:"; rlevel "Receive trigger level:"; ctsmode "Enable auto RTS/CTS"; addr "Base address:"
      mask help:
      | Diamond Emerald-MM
      | Serial
      | Setup
      mask init:
      | addr = hex2dec( addr(3:end) );
      mask Help: helpview(fullfile(docroot, 'mapfiles', 'xpc.map'), 'Baseboard_Setup')
      mask StyleString: popup(115200|57600|38400|19200|9600|4800|2400|1200|600|300|110),popup(5|6|7|8),popup(1|2),popup(None|Even|Odd|Mark|Space),popup(64 deep|16 deep|1 deep),popup(1|quarter full|half full|almost full),checkbox,edit,edit
      mask Display: disp('Diamond\nEmerald-MM8\nSetup');
  Write HW FIFO : S-Function  FunctionName=serwriteemeraldmm  Parameters=addr  mask(Write Data Port){addr=-1}
      mask prompts: addr "Base address:"
      mask help:
      | Diamond Emerald-MM
      | Write Data Port
      mask init:
      | addr = hex2dec( addr(3:end) );
      mask Help: helpview(fullfile(docroot, 'mapfiles', 'xpc.map'), 'Baseboard_Write_HW')
      mask Display:
      | disp('Diamond\nEmerald-MM8\nWrite Data Port');
      | port_label('input', 1, 'D');
      | port_label('input', 2, 'E');

== system xpclib/RS232/Mainboard/Baseboard Serial/RS232 ISR ==
  Xmt 1 : Inport  LatchInput=off
  Xmt 2 : Inport  Port=2  LatchInput=off
  function : TriggerPort  TriggerType=function-call
  While Iterator Subsystem : Subsystem  TreatAsAtomicUnit=on  PropExecContextAcrossSSBoundary=on
  Recv 1 : Outport
  Recv 2 : Outport  Port=2
  wires:
  Xmt 1/1 -> While Iterator Subsystem/1(Xmt 1)
  Xmt 2/1 -> While Iterator Subsystem/2(Xmt 2)
  While Iterator Subsystem/1(Recv 1) -> Recv 1/1
  While Iterator Subsystem/2(Recv 2) -> Recv 2/1

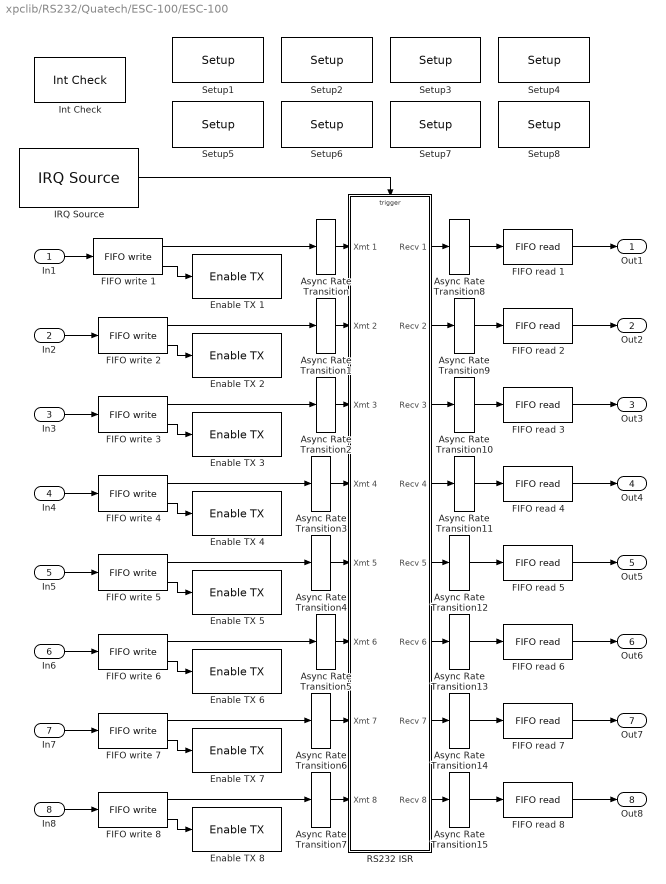
== system xpclib/RS232/Quatech/ESC-100/ESC-100 ==
  In1 : Inport  LatchInput=off
  In2 : Inport  Port=2  LatchInput=off
  In3 : Inport  Port=3  LatchInput=off
  In4 : Inport  Port=4  LatchInput=off
  In5 : Inport  Port=5  LatchInput=off
  In6 : Inport  Port=6  LatchInput=off
  In7 : Inport  Port=7  LatchInput=off
  In8 : Inport  Port=8  LatchInput=off
  Async Rate Transition{,1..15} (16 alike) : xpclib/Asynchronous Event/Async Rate Transition  sample_time=-1
  Enable TX 1 : xpclib/RS232/Quatech/ESC-100/ESC-100 Internal blocks/Enable TX   port=1  slot=brdslot
  Enable TX 2 : xpclib/RS232/Quatech/ESC-100/ESC-100 Internal blocks/Enable TX   port=2  slot=brdslot
  Enable TX 3 : xpclib/RS232/Quatech/ESC-100/ESC-100 Internal blocks/Enable TX   port=3  slot=brdslot
  Enable TX 4 : xpclib/RS232/Quatech/ESC-100/ESC-100 Internal blocks/Enable TX   port=4  slot=brdslot
  Enable TX 5 : xpclib/RS232/Quatech/ESC-100/ESC-100 Internal blocks/Enable TX   port=5  slot=brdslot
  Enable TX 6 : xpclib/RS232/Quatech/ESC-100/ESC-100 Internal blocks/Enable TX   port=6  slot=brdslot
  Enable TX 7 : xpclib/RS232/Quatech/ESC-100/ESC-100 Internal blocks/Enable TX   port=7  slot=brdslot
  Enable TX 8 : xpclib/RS232/Quatech/ESC-100/ESC-100 Internal blocks/Enable TX   port=8  slot=brdslot
  FIFO read {1..8} (8 alike) : xpclib/RS232/FIFO read   maxsize=1024  minsize=1  usedelimiter=on  delimiter=13  outputtype=count+16 bit uint  enable=off  enableout=off  sampletime=-1
  FIFO write 1 : xpclib/RS232/FIFO write   size=1024  inputtype=8 bit uint null terminated  present=on  sampletime=-1  id=XMT channel 1, IRQ 7
  FIFO write 2 : xpclib/RS232/FIFO write   size=1024  inputtype=8 bit uint null terminated  present=on  sampletime=-1  id=XMT channel 2, IRQ 7
  FIFO write 3 : xpclib/RS232/FIFO write   size=1024  inputtype=8 bit uint null terminated  present=on  sampletime=-1  id=XMT channel 3, IRQ 7
  FIFO write 4 : xpclib/RS232/FIFO write   size=1024  inputtype=8 bit uint null terminated  present=on  sampletime=-1  id=XMT channel 4, IRQ 7
  FIFO write 5 : xpclib/RS232/FIFO write   size=1024  inputtype=8 bit uint null terminated  present=on  sampletime=-1  id=XMT channel 5, IRQ 7
  FIFO write 6 : xpclib/RS232/FIFO write   size=1024  inputtype=8 bit uint null terminated  present=on  sampletime=-1  id=XMT channel 6, IRQ 7
  FIFO write 7 : xpclib/RS232/FIFO write   size=1024  inputtype=8 bit uint null terminated  present=on  sampletime=-1  id=XMT channel 7, IRQ 7
  FIFO write 8 : xpclib/RS232/FIFO write   size=1024  inputtype=8 bit uint null terminated  present=on  sampletime=-1  id=XMT channel 8, IRQ 7
  IRQ Source : xpclib/Asynchronous Event/IRQ Source  irqNo=7  preempt=off  b_type=None/Other  slot=brdslot
  Int Check : xpclib/RS232/Quatech/ESC-100/ESC-100 Internal blocks/Int Check  slot=brdslot  irqnum=7
  RS232 ISR : Subsystem  TreatAsAtomicUnit=on  PropExecContextAcrossSSBoundary=on  mask(RS232 ISR){slot=brdslot}
      mask help:
      | ESC-100
      | Quatech
      | Interrupt Service Routine
      mask init:
      | subslot = slot;
      mask Display:
      | disp('ESC-100\nISR');
      | port_label('input', 1, 'XMT1');
      | port_label('input', 2, 'XMT2');
      | port_label('input', 3, 'XMT3');
      | port_label('input', 4, 'XMT4');
      | port_label('input', 5, 'XMT5');
      | port_label('input', 6, 'XMT6');
      | port_label('input', 7, 'XMT7');
      | port_label('input', 8, 'XMT8');
      | port_label('output', 1, 'RCV1');
      | port_label('output', 2, 'RCV2');
      | port_label('output', 3, 'RCV3');
      | port_label('output', 4, 'RCV4');
      | port_label('output', 5, 'RCV5');
      | port_label('output', 6, 'RCV6');
      | port_label('output', 7, 'RCV7');
      | port_label('output', 8, 'RCV8');
  Setup1 : xpclib/RS232/Quatech/ESC-100/ESC-100 Internal blocks/Setup  port=1  baud=19200  width=8  nstop=1  parity=None  fmode=64 deep  rlevel=half full  ctsmode=on  slot=brdslot
  Setup2 : xpclib/RS232/Quatech/ESC-100/ESC-100 Internal blocks/Setup  port=2  baud=19200  width=8  nstop=1  parity=None  fmode=64 deep  rlevel=half full  ctsmode=on  slot=brdslot
  Setup3 : xpclib/RS232/Quatech/ESC-100/ESC-100 Internal blocks/Setup  port=3  baud=19200  width=8  nstop=1  parity=None  fmode=64 deep  rlevel=half full  ctsmode=on  slot=brdslot
  Setup4 : xpclib/RS232/Quatech/ESC-100/ESC-100 Internal blocks/Setup  port=4  baud=19200  width=8  nstop=1  parity=None  fmode=64 deep  rlevel=half full  ctsmode=on  slot=brdslot
  Setup5 : xpclib/RS232/Quatech/ESC-100/ESC-100 Internal blocks/Setup  port=5  baud=19200  width=8  nstop=1  parity=None  fmode=64 deep  rlevel=half full  ctsmode=on  slot=brdslot
  Setup6 : xpclib/RS232/Quatech/ESC-100/ESC-100 Internal blocks/Setup  port=6  baud=19200  width=8  nstop=1  parity=None  fmode=64 deep  rlevel=half full  ctsmode=on  slot=brdslot
  Setup7 : xpclib/RS232/Quatech/ESC-100/ESC-100 Internal blocks/Setup  port=7  baud=19200  width=8  nstop=1  parity=None  fmode=64 deep  rlevel=half full  ctsmode=on  slot=brdslot
  Setup8 : xpclib/RS232/Quatech/ESC-100/ESC-100 Internal blocks/Setup  port=8  baud=19200  width=8  nstop=1  parity=None  fmode=64 deep  rlevel=half full  ctsmode=on  slot=brdslot
  Out1 : Outport
  Out2 : Outport  Port=2
  Out3 : Outport  Port=3
  Out4 : Outport  Port=4
  Out5 : Outport  Port=5
  Out6 : Outport  Port=6
  Out7 : Outport  Port=7
  Out8 : Outport  Port=8
  wires:
  RS232 ISR/8(Recv 8) -> Async Rate Transition15/1
  RS232 ISR/7(Recv 7) -> Async Rate Transition14/1
  RS232 ISR/6(Recv 6) -> Async Rate Transition13/1
  RS232 ISR/5(Recv 5) -> Async Rate Transition12/1
  Async Rate Transition15/1 -> FIFO read 8/1
  FIFO read 8/1 -> Out8/1
  Async Rate Transition14/1 -> FIFO read 7/1
  FIFO read 7/1 -> Out7/1
  Async Rate Transition13/1 -> FIFO read 6/1
  FIFO read 6/1 -> Out6/1
  Async Rate Transition12/1 -> FIFO read 5/1
  FIFO read 5/1 -> Out5/1
  Async Rate Transition4/1 -> RS232 ISR/5(Xmt 5)
  Async Rate Transition5/1 -> RS232 ISR/6(Xmt 6)
  Async Rate Transition6/1 -> RS232 ISR/7(Xmt 7)
  Async Rate Transition7/1 -> RS232 ISR/8(Xmt 8)
  RS232 ISR/4(Recv 4) -> Async Rate Transition11/1
  Async Rate Transition1/1 -> RS232 ISR/2(Xmt 2)
  Async Rate Transition11/1 -> FIFO read 4/1
  Async Rate Transition10/1 -> FIFO read 3/1
  FIFO read 4/1 -> Out4/1
  FIFO read 3/1 -> Out3/1
  FIFO read 2/1 -> Out2/1
  Async Rate Transition9/1 -> FIFO read 2/1
  FIFO read 1/1 -> Out1/1
  Async Rate Transition8/1 -> FIFO read 1/1
  RS232 ISR/3(Recv 3) -> Async Rate Transition10/1
  RS232 ISR/2(Recv 2) -> Async Rate Transition9/1
  RS232 ISR/1(Recv 1) -> Async Rate Transition8/1
  Async Rate Transition3/1 -> RS232 ISR/4(Xmt 4)
  Async Rate Transition2/1 -> RS232 ISR/3(Xmt 3)
  Async Rate Transition/1 -> RS232 ISR/1(Xmt 1)
  IRQ Source/1 -> RS232 ISR/Trigger
  In1/1 -> FIFO write 1/1
  FIFO write 1/1 -> Async Rate Transition/1
  FIFO write 1/2 -> Enable TX 1/1
  FIFO write 2/1 -> Async Rate Transition1/1
  FIFO write 3/1 -> Async Rate Transition2/1
  FIFO write 4/1 -> Async Rate Transition3/1
  FIFO write 5/1 -> Async Rate Transition4/1
  FIFO write 6/1 -> Async Rate Transition5/1
  FIFO write 7/1 -> Async Rate Transition6/1
  FIFO write 8/1 -> Async Rate Transition7/1
  FIFO write 2/2 -> Enable TX 2/1
  FIFO write 3/2 -> Enable TX 3/1
  FIFO write 4/2 -> Enable TX 4/1
  FIFO write 5/2 -> Enable TX 5/1
  FIFO write 6/2 -> Enable TX 6/1
  FIFO write 7/2 -> Enable TX 7/1
  FIFO write 8/2 -> Enable TX 8/1
  In2/1 -> FIFO write 2/1
  In3/1 -> FIFO write 3/1
  In4/1 -> FIFO write 4/1
  In5/1 -> FIFO write 5/1
  In6/1 -> FIFO write 6/1
  In7/1 -> FIFO write 7/1
  In8/1 -> FIFO write 8/1
